simulink model "SF051A_SnsrOffsLrng"  (R2013b)
settings: Solver=FixedStepDiscrete  SolverMode=SingleTasking  StartTime=0.0  StopTime=1  FixedStep=0.002  RelTol=1e-3
undefined symbols (not defined in the file): ARCHGLBPRM_10MILLISEC_SEC_F32, ARCHGLBPRM_2MILLISEC_SEC_F32, ARCHGLBPRM_2PI_ULS_F32, ARCHGLBPRM_FLOATZEROTHD_ULS_F32, ARCHGLBPRM_PIOVER180_ULS_F32, CNV100MICROSECTOMILLISEC_MILLISECPERCNT_F32, CNV100MICROSECTOSEC_SECPERCNT_F32, COVRAMTRXNIT_ULS_F32, HWAUTHYTHD_ULS_F32, HWTQLRNGSTSLRND_CNT_U08, HWTQLRNGSTSNEGOFFS_CNT_U08, HWTQLRNGSTSNOTLRND_CNT_U08, HWTQLRNGSTSPOSOFFS_CNT_U08, HWTQLRNGSTSZEROOFFS_CNT_U08, HWTQLRNGTMRHILIM_SEC_F32, IDYMTRX_ULS_F32, IVS10MS_ULSPERSEC_F32, LRNGFILTICON_ULS_F32, NvmGetErrSts1, ONE_ULS_F32, SnsrOffsLrnd, SnsrOffsLrngFctEna, SnsrOffsLrngHwAgLrngDrvgDstThd, SnsrOffsLrngHwAgLrngEna, SnsrOffsLrngHwAgLrngHwVelThd, SnsrOffsLrngHwAgLrngSysTqThd, SnsrOffsLrngHwAgLrngSysTqThdMed, SnsrOffsLrngHwAgLrngSysTqThdTrustd, SnsrOffsLrngHwAgLrngSysTqThdWide, SnsrOffsLrngHwAgLrngTi, SnsrOffsLrngHwAgLrngVehSpdThd, SnsrOffsLrngHwAgLrngYawOffsDbnd, SnsrOffsLrngHwAgLrngYawRateThd, SnsrOffsLrngHwAgOffsLim, SnsrOffsLrngHwTqLrngEna, SnsrOffsLrngHwTqLrngEnaTiThd, SnsrOffsLrngHwTqLrngHwAgDbnd, SnsrOffsLrngHwTqLrngHwAgThd, SnsrOffsLrngHwTqLrngHwTqThd, SnsrOffsLrngHwTqLrngHwTqZeroOffsThd, SnsrOffsLrngHwTqLrngHwVelThd, SnsrOffsLrngHwTqLrngMeasTi, SnsrOffsLrngHwTqLrngMeasTiScar, SnsrOffsLrngHwTqLrngSampleImbThd1, SnsrOffsLrngHwTqLrngSampleImbThd2, SnsrOffsLrngHwTqLrngSampleThd1, SnsrOffsLrngHwTqLrngSampleThd2, SnsrOffsLrngHwTqLrngTiWghtCoeff, SnsrOffsLrngHwTqLrngVehSpdThd, SnsrOffsLrngHwTqOffsLim, SnsrOffsLrngSampleCntForHwTqLrngRst, SnsrOffsLrngTqInpDetnPwrEstimnThd, SnsrOffsLrngTqInpDetnSinGenrAmp, SnsrOffsLrngTqInpDetnSinGenrFrq, SnsrOffsLrngTqInpDetnStg1FilGain, SnsrOffsLrngTqInpDetnStg1WinSize, SnsrOffsLrngTqInpDetnStg2FilGainCen, SnsrOffsLrngTqInpDetnStg2FilGainDwn, SnsrOffsLrngTqInpDetnStg2FilGainUp, SnsrOffsLrngTqInpDetnStg2WinSize ... (+15)
libraries: Fil x34, FixdToFloat x17, FloatToFixd x16, NxtrLim x15, simulink x12, NxtrAbslt x12, NxtrNvM x8, NxtrMin x5, NxtrMath x3
(part 5 of 11)

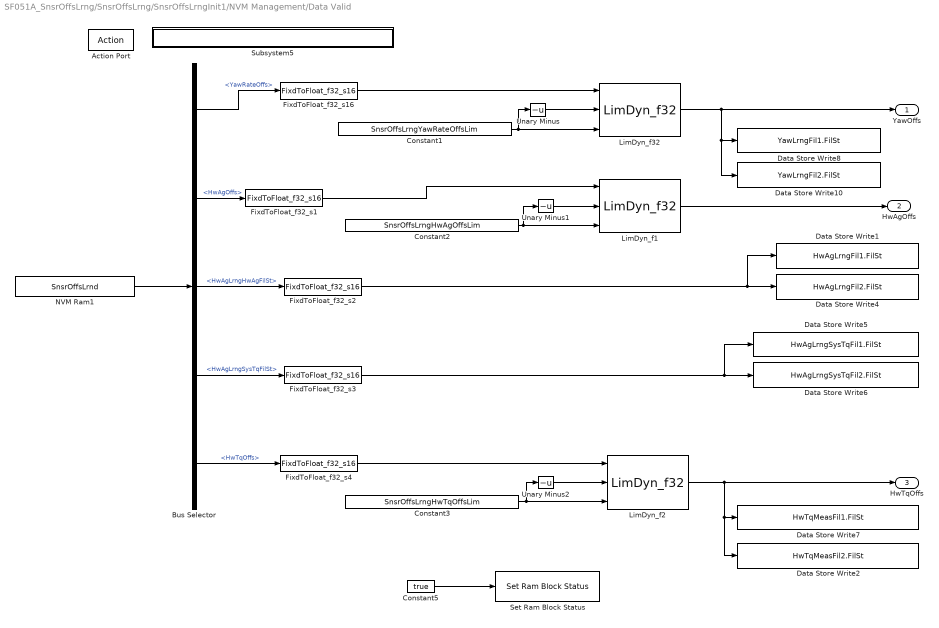
== system SF051A_SnsrOffsLrng/SnsrOffsLrng/SnsrOffsLrngInit1/NVM Management/Data Valid ==
  Action Port : ActionPort  ActionType=else
  Bus Selector : BusSelector  OutputSignals=YawRateOffs,HwAgOffs,HwAgLrngHwAgFilSt,HwAgLrngSysTqFilSt,HwTqOffs
  Constant1 : Constant  RequirementInfo={'linktype_rmi_doors' '0000babd (/E-STEER Core/SubSystem Specifications/Application Functions/SF051A Sensor Offset Learning)' '#SF051A_199' 'true' 'REQ:SF051A_199' '' } %GIDa_076ebffe_b680_48ef_8f96_8d7c4d22071c  Value=SnsrOffsLrngYawRateOffsLim  OutDataTypeStr=single
  Constant2 : Constant  RequirementInfo={'linktype_rmi_doors' '0000babd (/E-STEER Core/SubSystem Specifications/Application Functions/SF051A Sensor Offset Learning)' '#SF051A_200' 'true' 'REQ:SF051A_200' '' } %GIDa_86e1dd64_5744_4dce_ae9a_588dfe94c923  Value=SnsrOffsLrngHwAgOffsLim  OutDataTypeStr=single
  Constant3 : Constant  RequirementInfo={'linktype_rmi_doors' '0000babd (/E-STEER Core/SubSystem Specifications/Application Functions/SF051A Sensor Offset Learning)' '#SF051A_197' 'true' 'REQ:SF051A_197' '' } %GIDa_41a18de5_d6df_4abf_8798_f58c94a277e5  Value=SnsrOffsLrngHwTqOffsLim  OutDataTypeStr=single
  Constant5 : Constant  Value=true  OutDataTypeStr=boolean
      settings: AttributesFormatString=%<OutDataTypeStr>
  Data Store Write1 : DataStoreWrite  DataStoreName=HwAgLrngFil1  DataStoreElements=HwAgLrngFil1.FilSt
  Data Store Write10 : DataStoreWrite  DataStoreName=YawLrngFil2  DataStoreElements=YawLrngFil2.FilSt
  Data Store Write2 : DataStoreWrite  DataStoreName=HwTqMeasFil2  DataStoreElements=HwTqMeasFil2.FilSt
  Data Store Write4 : DataStoreWrite  DataStoreName=HwAgLrngFil2  DataStoreElements=HwAgLrngFil2.FilSt
  Data Store Write5 : DataStoreWrite  DataStoreName=HwAgLrngSysTqFil1  DataStoreElements=HwAgLrngSysTqFil1.FilSt
  Data Store Write6 : DataStoreWrite  DataStoreName=HwAgLrngSysTqFil2  DataStoreElements=HwAgLrngSysTqFil2.FilSt
  Data Store Write7 : DataStoreWrite  DataStoreName=HwTqMeasFil1  DataStoreElements=HwTqMeasFil1.FilSt
  Data Store Write8 : DataStoreWrite  DataStoreName=YawLrngFil1  DataStoreElements=YawLrngFil1.FilSt
  FixdToFloat_f32_s1 : FixdToFloat/FixdToFloat_f32_s16  Param1=10
  FixdToFloat_f32_s16 : FixdToFloat/FixdToFloat_f32_s16  Param1=9
  FixdToFloat_f32_s2 : FixdToFloat/FixdToFloat_f32_s16  Param1=4
  FixdToFloat_f32_s3 : FixdToFloat/FixdToFloat_f32_s16  Param1=5
  FixdToFloat_f32_s4 : FixdToFloat/FixdToFloat_f32_s16  Param1=12
  LimDyn_f1 : NxtrLim/LimDyn_f32  RequirementInfo={'linktype_rmi_doors' '0000babd (/E-STEER Core/SubSystem Specifications/Application Functions/SF051A Sensor Offset Learning)' '#SF051A_200' 'true' 'REQ:SF051A_200' '' } %GIDa_a6942d9b_ce75_427e_8670_f0f4de9cc18b
  LimDyn_f2 : NxtrLim/LimDyn_f32  RequirementInfo={'linktype_rmi_doors' '0000babd (/E-STEER Core/SubSystem Specifications/Application Functions/SF051A Sensor Offset Learning)' '#SF051A_197' 'true' 'REQ:SF051A_197' '' } %GIDa_a3cd0533_6baf_48d9_892e_aa8de74fd927
  LimDyn_f32 : NxtrLim/LimDyn_f32  RequirementInfo={'linktype_rmi_doors' '0000babd (/E-STEER Core/SubSystem Specifications/Application Functions/SF051A Sensor Offset Learning)' '#SF051A_199' 'true' 'REQ:SF051A_199' '' } %GIDa_1308976f_16df_4360_a216_3c89b58824fa
  NVM Ram1 : DataStoreRead  DataStoreName=SnsrOffsLrnd
  Set Ram Block Status : NxtrNvM/Set Ram Block Status  FuncName=Set Ram Block Status  NvMBlockName=SnsrOffsLrnd  VoidFuncRtn=on  BlockChanged_DSN=NvMSRBS_BlockChanged2  Return_DSN=NvMSRBS_Return2
      settings: AttributesFormatString=%<FuncName>
  Subsystem5 : Subsystem  Description=|  mask(Copyright Information){none=on}
      | Copyright info block.                                               
      |                                                                     
      | Place copyright information at the top of every subsystem in design.
      mask prompts: none "No parameters"
      mask help: Place copyright information at the top of every subsystem in design.
      mask Display:
      | NxtrConf = 'Nexteer Confidential';
      | 
      | sys = bdroot; %handle for the current model ("system")
      | first = get_param(sys,'Created');
      | first = first(end-3:end);  %year is last four digits
      | 
      | last = get_param(sys,'LastModifiedDate');
      | if isempty(last)
      |     last = datestr(now,'yyyy');
      | else
      |     last = last(end-3:end);
      | end
      | 
      | if strcmp(first,last)
      |     fprintf('%s -- Copyright %s Nexteer',NxtrConf,first)
      | else
      |     fprintf('%s -- %s%s- %s Nexteer',NxtrConf,char(169),first,last)
      | end
  Unary Minus : UnaryMinus  RequirementInfo={'linktype_rmi_doors' '0000babd (/E-STEER Core/SubSystem Specifications/Application Functions/SF051A Sensor Offset Learning)' '#SF051A_199' 'true' 'REQ:SF051A_199' '' } %GIDa_10d4a236_00c8_44d2_88c9_a38d910bd610
  Unary Minus1 : UnaryMinus  RequirementInfo={'linktype_rmi_doors' '0000babd (/E-STEER Core/SubSystem Specifications/Application Functions/SF051A Sensor Offset Learning)' '#SF051A_200' 'true' 'REQ:SF051A_200' '' } %GIDa_5c1b3055_1216_4150_a142_355401d5d7f1
  Unary Minus2 : UnaryMinus  RequirementInfo={'linktype_rmi_doors' '0000babd (/E-STEER Core/SubSystem Specifications/Application Functions/SF051A Sensor Offset Learning)' '#SF051A_197' 'true' 'REQ:SF051A_197' '' } %GIDa_8a9aa98b_e7a9_4fa6_add4_1fe4b896ad88
  YawOffs : Outport
  HwAgOffs : Outport  Port=2
  HwTqOffs : Outport  Port=3
  wires:
  NVM Ram1/1 -> Bus Selector/1
  Bus Selector/1 -> FixdToFloat_f32_s16/1  "<YawRateOffs>"
  Bus Selector/2 -> FixdToFloat_f32_s1/1  "<HwAgOffs>"
  Bus Selector/5 -> FixdToFloat_f32_s4/1  "<HwTqOffs>"
  Constant1/1 -> LimDyn_f32/3, Unary Minus/1
  LimDyn_f32/1 -> YawOffs/1, Data Store Write8/1, Data Store Write10/1
  Constant2/1 -> Unary Minus1/1, LimDyn_f1/3
  Constant3/1 -> Unary Minus2/1, LimDyn_f2/3
  LimDyn_f2/1 -> Data Store Write2/1, Data Store Write7/1, HwTqOffs/1
  Bus Selector/4 -> FixdToFloat_f32_s3/1  "<HwAgLrngSysTqFilSt>"
  Bus Selector/3 -> FixdToFloat_f32_s2/1  "<HwAgLrngHwAgFilSt>"
  Constant5/1 -> Set Ram Block Status/1
  FixdToFloat_f32_s2/1 -> Data Store Write1/1, Data Store Write4/1
  FixdToFloat_f32_s3/1 -> Data Store Write5/1, Data Store Write6/1
  Unary Minus/1 -> LimDyn_f32/2
  Unary Minus2/1 -> LimDyn_f2/2
  FixdToFloat_f32_s4/1 -> LimDyn_f2/1
  FixdToFloat_f32_s16/1 -> LimDyn_f32/1
  LimDyn_f1/1 -> HwAgOffs/1
  Unary Minus1/1 -> LimDyn_f1/2
  FixdToFloat_f32_s1/1 -> LimDyn_f1/1

== system SF051A_SnsrOffsLrng/SnsrOffsLrng/SnsrOffsLrngInit1/NVM Management/Not Enabled ==
  note: The entire function has been disabled via one boolean calibration.  Output zeros
      | and tell Nvm Mgr not to bother writing Nvm values at key off.
  Action Port : ActionPort  ActionType=then
  Constant : Constant  RequirementInfo={'linktype_rmi_doors' '0000babd (/E-STEER Core/SubSystem Specifications/Application Functions/SF051A Sensor Offset Learning)' '#SF051A_244' 'true' 'REQ:SF051A_244' '' ; 'linktype_rmi_doors' '0000babd (/E-STEER Core/SubSystem Specifications/Application Functions/SF051A Sensor Offset Learning)' '#SF051A_245' 'true' 'REQ:SF051A_245' '' ; 'linktype_rmi_doors' '0000babd (/E-STEER Core/SubSystem Specifications/Application Functions/SF051A Sensor Offset Learning)' '#SF051A_45' 'true' 'REQ:SF051A_45' '' } %GIDa_7bd904ef_6dfb_4655_9af9_edb8e6d91ac1  Value=ZERO_ULS_F32  OutDataTypeStr=single
      settings: AttributesFormatString=%<OutDataTypeStr>
  Subsystem5 : Subsystem  Description=|  mask(Copyright Information){none=on}
      | Copyright info block.                                               
      |                                                                     
      | Place copyright information at the top of every subsystem in design.
      mask prompts: none "No parameters"
      mask help: Place copyright information at the top of every subsystem in design.
      mask Display:
      | NxtrConf = 'Nexteer Confidential';
      | 
      | sys = bdroot; %handle for the current model ("system")
      | first = get_param(sys,'Created');
      | first = first(end-3:end);  %year is last four digits
      | 
      | last = get_param(sys,'LastModifiedDate');
      | if isempty(last)
      |     last = datestr(now,'yyyy');
      | else
      |     last = last(end-3:end);
      | end
      | 
      | if strcmp(first,last)
      |     fprintf('%s -- Copyright %s Nexteer',NxtrConf,first)
      | else
      |     fprintf('%s -- %s%s- %s Nexteer',NxtrConf,char(169),first,last)
      | end
  YawOffs : Outport  RequirementInfo={'linktype_rmi_doors' '0000babd (/E-STEER Core/SubSystem Specifications/Application Functions/SF051A Sensor Offset Learning)' '#SF051A_244' 'true' 'REQ:SF051A_244' '' } %GIDa_19bbba3b_0dec_46be_8ce3_0daa8b4bfd81
  HwAgOffs : Outport  RequirementInfo={'linktype_rmi_doors' '0000babd (/E-STEER Core/SubSystem Specifications/Application Functions/SF051A Sensor Offset Learning)' '#SF051A_245' 'true' 'REQ:SF051A_245' '' } %GIDa_7ded515a_2b55_49df_86d7_0efec96a218f  Port=2
  HwTqOffs : Outport  RequirementInfo={'linktype_rmi_doors' '0000babd (/E-STEER Core/SubSystem Specifications/Application Functions/SF051A Sensor Offset Learning)' '#SF051A_45' 'true' 'REQ:SF051A_45' '' } %GIDa_401e0381_36a7_4d73_9c61_1f70a1280659  Port=3
  wires:
  Constant/1 -> HwTqOffs/1, HwAgOffs/1, YawOffs/1

== system SF051A_SnsrOffsLrng/SnsrOffsLrng/SnsrOffsLrngInit1/NVM Management/Subsystem5 ==

== system SF051A_SnsrOffsLrng/SnsrOffsLrng/SnsrOffsLrngPer1/EnableLearning/Default_TqInpDetn ==
  Action Port : ActionPort  ActionType=else
  Constant : Constant  Value=false  OutDataTypeStr=boolean
      settings: AttributesFormatString=%<OutDataTypeStr>
  Constant1 : Constant  Value=true  OutDataTypeStr=boolean
      settings: AttributesFormatString=%<OutDataTypeStr>
  Subsystem5 : Subsystem  Description=|  mask(Copyright Information){none=on}
      | Copyright info block.                                               
      |                                                                     
      | Place copyright information at the top of every subsystem in design.
      mask prompts: none "No parameters"
      mask help: Place copyright information at the top of every subsystem in design.
      mask Display:
      | NxtrConf = 'Nexteer Confidential';
      | 
      | sys = bdroot; %handle for the current model ("system")
      | first = get_param(sys,'Created');
      | first = first(end-3:end);  %year is last four digits
      | 
      | last = get_param(sys,'LastModifiedDate');
      | if isempty(last)
      |     last = datestr(now,'yyyy');
      | else
      |     last = last(end-3:end);
      | end
      | 
      | if strcmp(first,last)
      |     fprintf('%s -- Copyright %s Nexteer',NxtrConf,first)
      | else
      |     fprintf('%s -- %s%s- %s Nexteer',NxtrConf,char(169),first,last)
      | end
  TqInpPresVld : Outport  InitialOutput=0
  TqInpPrsnt : Outport  Port=2  InitialOutput=0
  wires:
  Constant1/1 -> TqInpPrsnt/1  "TqInpPrsnt"
  Constant/1 -> TqInpPresVld/1  "TqInpPresVld"

== system SF051A_SnsrOffsLrng/SnsrOffsLrng/SnsrOffsLrngPer1/EnableLearning/EnablingConditions ==
  note: Prevents to keep taking the same measurements once again
      | again if the handwheel didn't chaged its position
  note: Limits the HwPos range that will be used for the learning.
      | defined by the Learning algorithm
  note: Vehicle speed need to be 0 kph in order to get less noisy
      | measurements. It is also the situation when it is most probable
      | to find a NoTorqueInputPresent situation.
  note: Handwheel need to be stopped.
  note: Handwheel torque needs to be close to zero.. This claibration
      | cannot have the same value than the maximum HwTrq that
      | will be stored (Learning algotihm needs HwTrq values out of that
      | range in order to work).
  HwTq : Inport
  HwVel : Inport  Port=2
  VehSpd : Inport  Port=3
  HwAg : Inport  Port=4
  Abslt_f32_f1 : NxtrAbslt/Abslt_f32_f32  RequirementInfo={'linktype_rmi_doors' '0000babd (/E-STEER Core/SubSystem Specifications/Application Functions/SF051A Sensor Offset Learning)' '#SF051A_164' 'true' 'REQ:SF051A_164' '' } %GIDa_9e6654fc_c12f_4f0b_b95d_e68a683dad8f  SFunctionSpec=single y1 = Abslt_f32_f32(single u1)
      settings: AttributesFormatString=%<Name>
  Abslt_f32_f2 : NxtrAbslt/Abslt_f32_f32  RequirementInfo={'linktype_rmi_doors' '0000babd (/E-STEER Core/SubSystem Specifications/Application Functions/SF051A Sensor Offset Learning)' '#SF051A_164' 'true' 'REQ:SF051A_164' '' } %GIDa_f22554bc_685a_43e5_b318_a11f967165d9  SFunctionSpec=single y1 = Abslt_f32_f32(single u1)
      settings: AttributesFormatString=%<Name>
  Abslt_f32_f32 : NxtrAbslt/Abslt_f32_f32  RequirementInfo={'linktype_rmi_doors' '0000babd (/E-STEER Core/SubSystem Specifications/Application Functions/SF051A Sensor Offset Learning)' '#SF051A_164' 'true' 'REQ:SF051A_164' '' } %GIDa_e92dafa2_36c7_4571_935e_c15c4f7f6a46  SFunctionSpec=single y1 = Abslt_f32_f32(single u1)
      settings: AttributesFormatString=%<Name>
  CheckLastMeasHwPos : Subsystem  RequirementInfo={'linktype_rmi_doors' '0000babd (/E-STEER Core/SubSystem Specifications/Application Functions/SF051A Sensor Offset Learning)' '#SF051A_153' 'true' 'REQ:SF051A_153' '' } %GIDa_44e6e44d_9c2d_4a29_b17b_bdb322509a04
  Constant : Constant  RequirementInfo={'linktype_rmi_doors' '0000babd (/E-STEER Core/SubSystem Specifications/Application Functions/SF051A Sensor Offset Learning)' '#SF051A_164' 'true' 'REQ:SF051A_164' '' } %GIDa_78b0b28d_512c_4bbe_9a88_b290db340ca2  Value=SnsrOffsLrngHwTqLrngHwTqThd
  Constant1 : Constant  RequirementInfo={'linktype_rmi_doors' '0000babd (/E-STEER Core/SubSystem Specifications/Application Functions/SF051A Sensor Offset Learning)' '#SF051A_164' 'true' 'REQ:SF051A_164' '' } %GIDa_6cae68dc_855b_480e_9fca_bfbaa07e5595  Value=SnsrOffsLrngHwTqLrngHwVelThd
  Constant2 : Constant  RequirementInfo={'linktype_rmi_doors' '0000babd (/E-STEER Core/SubSystem Specifications/Application Functions/SF051A Sensor Offset Learning)' '#SF051A_164' 'true' 'REQ:SF051A_164' '' } %GIDa_db8aa412_af43_4293_866b_dc91b376e004  Value=SnsrOffsLrngHwTqLrngVehSpdThd
  Constant3 : Constant  RequirementInfo={'linktype_rmi_doors' '0000babd (/E-STEER Core/SubSystem Specifications/Application Functions/SF051A Sensor Offset Learning)' '#SF051A_164' 'true' 'REQ:SF051A_164' '' } %GIDa_56d7e85f_b29d_46f1_86ec_479da9e5d3a2  Value=SnsrOffsLrngHwTqLrngHwAgThd
  Logical Operator : Logic  RequirementInfo={'linktype_rmi_doors' '0000babd (/E-STEER Core/SubSystem Specifications/Application Functions/SF051A Sensor Offset Learning)' '#SF051A_164' 'true' 'REQ:SF051A_164' '' ; 'linktype_rmi_doors' '0000babd (/E-STEER Core/SubSystem Specifications/Application Functions/SF051A Sensor Offset Learning)' '#SF051A_153' 'true' 'REQ:SF051A_153' '' } %GIDa_67f5e3c6_c811_4f06_9205_8d434655c309  Inputs=5  AllPortsSameDT=off  OutDataTypeStr=boolean
  Relational Operator : RelationalOperator  RequirementInfo={'linktype_rmi_doors' '0000babd (/E-STEER Core/SubSystem Specifications/Application Functions/SF051A Sensor Offset Learning)' '#SF051A_164' 'true' 'REQ:SF051A_164' '' } %GIDa_64107afe_b0ad_4ff5_abd5_e1ad1dd60b07  Operator=<=  OutDataTypeStr=boolean
  Relational Operator1 : RelationalOperator  RequirementInfo={'linktype_rmi_doors' '0000babd (/E-STEER Core/SubSystem Specifications/Application Functions/SF051A Sensor Offset Learning)' '#SF051A_164' 'true' 'REQ:SF051A_164' '' } %GIDa_a80d4eac_68b4_4a5c_93ef_0c10081c4193  Operator=<=  OutDataTypeStr=boolean
  Relational Operator2 : RelationalOperator  RequirementInfo={'linktype_rmi_doors' '0000babd (/E-STEER Core/SubSystem Specifications/Application Functions/SF051A Sensor Offset Learning)' '#SF051A_164' 'true' 'REQ:SF051A_164' '' } %GIDa_b1b96eb6_2e47_4324_bb24_5b2841330fb5  Operator=<=  OutDataTypeStr=boolean
  Relational Operator3 : RelationalOperator  RequirementInfo={'linktype_rmi_doors' '0000babd (/E-STEER Core/SubSystem Specifications/Application Functions/SF051A Sensor Offset Learning)' '#SF051A_164' 'true' 'REQ:SF051A_164' '' } %GIDa_3484eb6c_a506_422c_9fce_52f4631db782  Operator=<=  OutDataTypeStr=boolean
  Subsystem5 : Subsystem  Description=|  mask(Copyright Information){none=on}
      | Copyright info block.                                               
      |                                                                     
      | Place copyright information at the top of every subsystem in design.
      mask prompts: none "No parameters"
      mask help: Place copyright information at the top of every subsystem in design.
      mask Display:
      | NxtrConf = 'Nexteer Confidential';
      | 
      | sys = bdroot; %handle for the current model ("system")
      | first = get_param(sys,'Created');
      | first = first(end-3:end);  %year is last four digits
      | 
      | last = get_param(sys,'LastModifiedDate');
      | if isempty(last)
      |     last = datestr(now,'yyyy');
      | else
      |     last = last(end-3:end);
      | end
      | 
      | if strcmp(first,last)
      |     fprintf('%s -- Copyright %s Nexteer',NxtrConf,first)
      | else
      |     fprintf('%s -- %s%s- %s Nexteer',NxtrConf,char(169),first,last)
      | end
  TqInpDetnEna : Outport
  wires:
  CheckLastMeasHwPos/1(HwAgMoved) -> Logical Operator/5
  Abslt_f32_f2/1 -> Relational Operator3/1
  Constant3/1 -> Relational Operator3/2
  VehSpd/1 -> Relational Operator2/1
  Constant2/1 -> Relational Operator2/2
  Abslt_f32_f1/1 -> Relational Operator1/1
  Constant1/1 -> Relational Operator1/2
  Constant/1 -> Relational Operator/2
  Abslt_f32_f32/1 -> Relational Operator/1
  Relational Operator3/1 -> Logical Operator/4
  HwAg/1 -> Abslt_f32_f2/1, CheckLastMeasHwPos/1(HwAg)
  Logical Operator/1 -> TqInpDetnEna/1  "TqInpDetnEna"
  Relational Operator1/1 -> Logical Operator/2
  HwVel/1 -> Abslt_f32_f1/1
  HwTq/1 -> Abslt_f32_f32/1
  Relational Operator2/1 -> Logical Operator/3
  Relational Operator/1 -> Logical Operator/1

== system SF051A_SnsrOffsLrng/SnsrOffsLrng/SnsrOffsLrngPer1/EnableLearning/Eval_Time ==
  note: In MilliSec
  Action Port : ActionPort  ActionType=then
  100MicroSecToMilliSec : Constant  Value=CNV100MICROSECTOMILLISEC_MILLISECPERCNT_F32
  Constant : Constant  Value=SnsrOffsLrngHwTqLrngEnaTiThd
  Data Store Read : DataStoreRead  DataStoreName=HwTqLrngEnaTmrRef
  FixdToFloat_f32_u32 : FixdToFloat/FixdToFloat_f32_u32  Param1=0
  GetTiSpan100MicroSec32bit : Subsystem  mask(Timer_GTS){}
      mask help: Used to get the time span between start and current time.
  Product : Product
  Relational Operator : RelationalOperator  OutDataTypeStr=boolean
  Subsystem5 : Subsystem  Description=|  mask(Copyright Information){none=on}
      | Copyright info block.                                               
      |                                                                     
      | Place copyright information at the top of every subsystem in design.
      mask prompts: none "No parameters"
      mask help: Place copyright information at the top of every subsystem in design.
      mask Display:
      | NxtrConf = 'Nexteer Confidential';
      | 
      | sys = bdroot; %handle for the current model ("system")
      | first = get_param(sys,'Created');
      | first = first(end-3:end);  %year is last four digits
      | 
      | last = get_param(sys,'LastModifiedDate');
      | if isempty(last)
      |     last = datestr(now,'yyyy');
      | else
      |     last = last(end-3:end);
      | end
      | 
      | if strcmp(first,last)
      |     fprintf('%s -- Copyright %s Nexteer',NxtrConf,first)
      | else
      |     fprintf('%s -- %s%s- %s Nexteer',NxtrConf,char(169),first,last)
      | end
  HwTqLrngEna : Outport
  wires:
  Data Store Read/1 -> GetTiSpan100MicroSec32bit/1(RefTmr)
  Constant/1 -> Relational Operator/2
  Relational Operator/1 -> HwTqLrngEna/1
  GetTiSpan100MicroSec32bit/1(TiSpan) -> FixdToFloat_f32_u32/1
  Product/1 -> Relational Operator/1
  100MicroSecToMilliSec/1 -> Product/2
  FixdToFloat_f32_u32/1 -> Product/1

== system SF051A_SnsrOffsLrng/SnsrOffsLrng/SnsrOffsLrngPer1/EnableLearning/False_Reset ==
  Action Port : ActionPort  ActionType=else
  Constant : Constant  Value=false  OutDataTypeStr=boolean
      settings: AttributesFormatString=%<OutDataTypeStr>
  Data Store Write : DataStoreWrite  DataStoreName=HwTqLrngEnaTmrRef
  GetRefTmr100MicroSec32bit : Subsystem
  Subsystem5 : Subsystem  Description=|  mask(Copyright Information){none=on}
      | Copyright info block.                                               
      |                                                                     
      | Place copyright information at the top of every subsystem in design.
      mask prompts: none "No parameters"
      mask help: Place copyright information at the top of every subsystem in design.
      mask Display:
      | NxtrConf = 'Nexteer Confidential';
      | 
      | sys = bdroot; %handle for the current model ("system")
      | first = get_param(sys,'Created');
      | first = first(end-3:end);  %year is last four digits
      | 
      | last = get_param(sys,'LastModifiedDate');
      | if isempty(last)
      |     last = datestr(now,'yyyy');
      | else
      |     last = last(end-3:end);
      | end
      | 
      | if strcmp(first,last)
      |     fprintf('%s -- Copyright %s Nexteer',NxtrConf,first)
      | else
      |     fprintf('%s -- %s%s- %s Nexteer',NxtrConf,char(169),first,last)
      | end
  HwTqLrngEna : Outport
  wires:
  Constant/1 -> HwTqLrngEna/1
  GetRefTmr100MicroSec32bit/1(RefTmr) -> Data Store Write/1

== system SF051A_SnsrOffsLrng/SnsrOffsLrng/SnsrOffsLrngPer1/EnableLearning/Filter_HwTq ==
  HwTq : Inport
  Display : DataStoreWrite  DataStoreName=dSnsrOffsLrngTqInpDetnHwTqFild
  FilLpUpdOutp : Fil/FilLpUpdOutp  StVar=TqInpDetnHwTqFil
      settings: AttributesFormatString=StVar: %<StVar>
  Subsystem5 : Subsystem  Description=|  mask(Copyright Information){none=on}
      | Copyright info block.                                               
      |                                                                     
      | Place copyright information at the top of every subsystem in design.
      mask prompts: none "No parameters"
      mask help: Place copyright information at the top of every subsystem in design.
      mask Display:
      | NxtrConf = 'Nexteer Confidential';
      | 
      | sys = bdroot; %handle for the current model ("system")
      | first = get_param(sys,'Created');
      | first = first(end-3:end);  %year is last four digits
      | 
      | last = get_param(sys,'LastModifiedDate');
      | if isempty(last)
      |     last = datestr(now,'yyyy');
      | else
      |     last = last(end-3:end);
      | end
      | 
      | if strcmp(first,last)
      |     fprintf('%s -- Copyright %s Nexteer',NxtrConf,first)
      | else
      |     fprintf('%s -- %s%s- %s Nexteer',NxtrConf,char(169),first,last)
      | end
  HwTqFild : Outport
  wires:
  HwTq/1 -> FilLpUpdOutp/1
  FilLpUpdOutp/1 -> Display/1, HwTqFild/1

== system SF051A_SnsrOffsLrng/SnsrOffsLrng/SnsrOffsLrngPer1/EnableLearning/Perform_TqInpDetn ==
  note: Reset may or may not happen, but if it does, it must happen before PreProcessing executes.
  note: Step 1
  note: Step 2
  HwTqFild : Inport
  TqInpDetnEnaPrev : Inport  Port=2
  Action Port : ActionPort  ActionType=then
  Do nothing : Subsystem  TreatAsAtomicUnit=on
  ElapsedTime : Subsystem  Priority=2
      settings: AttributesFormatString=Priority: %<Priority>
  Enable_PreProcessing : Subsystem  Priority=2  TreatAsAtomicUnit=on
      settings: AttributesFormatString=Priority: %<Priority>
  If1 : If  Priority=1  IfExpression=~u1
      settings: AttributesFormatString=Priority: %<Priority>
  SetStuffToZero : Subsystem  Priority=1  TreatAsAtomicUnit=on
      settings: AttributesFormatString=Priority: %<Priority>
  StateVariable : DataStoreWrite  Priority=2  DataStoreName=HwTqLrngTqInpPrsnt
      settings: AttributesFormatString=Priority: %<Priority>
  Subsystem5 : Subsystem  Description=|  mask(Copyright Information){none=on}
      | Copyright info block.                                               
      |                                                                     
      | Place copyright information at the top of every subsystem in design.
      mask prompts: none "No parameters"
      mask help: Place copyright information at the top of every subsystem in design.
      mask Display:
      | NxtrConf = 'Nexteer Confidential';
      | 
      | sys = bdroot; %handle for the current model ("system")
      | first = get_param(sys,'Created');
      | first = first(end-3:end);  %year is last four digits
      | 
      | last = get_param(sys,'LastModifiedDate');
      | if isempty(last)
      |     last = datestr(now,'yyyy');
      | else
      |     last = last(end-3:end);
      | end
      | 
      | if strcmp(first,last)
      |     fprintf('%s -- Copyright %s Nexteer',NxtrConf,first)
      | else
      |     fprintf('%s -- %s%s- %s Nexteer',NxtrConf,char(169),first,last)
      | end
  TqInpPrsntVld : Outport  InitialOutput=0
  TqInpPrsnt : Outport  Port=2  InitialOutput=0
  wires:
  ElapsedTime/1(TiEnad) -> Enable_PreProcessing/1(TiEnad)
  Enable_PreProcessing/2(TqInpPrsnt) -> TqInpPrsnt/1, StateVariable/1  "TqInpPrsnt"
  Enable_PreProcessing/1(TqInpPrsntVld) -> TqInpPrsntVld/1  "TqInpPrsntVld"
  If1/1 -> SetStuffToZero/Action
  TqInpDetnEnaPrev/1 -> If1/1
  HwTqFild/1 -> Enable_PreProcessing/2(HwTqFild)
  If1/2 -> Do nothing/Action

== system SF051A_SnsrOffsLrng/SnsrOffsLrng/SnsrOffsLrngPer1/EnableLearning/Subsystem5 ==

== system SF051A_SnsrOffsLrng/SnsrOffsLrng/SnsrOffsLrngPer1/Hold/Subsystem5 ==

== system SF051A_SnsrOffsLrng/SnsrOffsLrng/SnsrOffsLrngPer1/Learning/CalculateOnCenterTorqueDrift ==
  note: The considered mathematical model HwTq vs HwAg follows:
      |                    Y = A*sin(X + Phi) + B
      | Where:
      | -. X = HwAg
      | -. Y = HwTq
      | -. A is the HwTq reading when Tq_Off=0Nm, Phi=0Deg and HwAg=90°
      | -. Phi = HwAg_Offset
      | -. B = HwTq_Offset
      |
      | That model can also be written as:
      |                Y = A1*sin(X) + A2*cos(X) + B
      | Where: A = sqrt(A1^2+A2^2)   and   sin(Phi) = A2/A
      |
      | The RLSE estimates the parameters A1, A2 and B, which are used to
      | calculate the HwTq Offset.
  note: In this version, the HwTq Offset is considered more specifically as the
      | HwTq drift for HwAg = 0Deg (OnCenter). Replacing in the mathematical
      | model:
      |                Y = A1*sin(0°) + A2*cos(0°) + B
      |                             Y = A2 + B
      | Therefore,
      |           HwTqOnCenterDrift = A2 + HwTq_Off
  HwTqOffsEstimd : Inport
  A2 : Inport  Port=2
  Add1 : Sum
  Display1 : DataStoreWrite  DataStoreName=dSnsrOffsLrngHwTqLrngHwTqOffsRaw
  Subsystem5 : Subsystem  Description=|  mask(Copyright Information){none=on}
      | Copyright info block.                                               
      |                                                                     
      | Place copyright information at the top of every subsystem in design.
      mask prompts: none "No parameters"
      mask help: Place copyright information at the top of every subsystem in design.
      mask Display:
      | NxtrConf = 'Nexteer Confidential';
      | 
      | sys = bdroot; %handle for the current model ("system")
      | first = get_param(sys,'Created');
      | first = first(end-3:end);  %year is last four digits
      | 
      | last = get_param(sys,'LastModifiedDate');
      | if isempty(last)
      |     last = datestr(now,'yyyy');
      | else
      |     last = last(end-3:end);
      | end
      | 
      | if strcmp(first,last)
      |     fprintf('%s -- Copyright %s Nexteer',NxtrConf,first)
      | else
      |     fprintf('%s -- %s%s- %s Nexteer',NxtrConf,char(169),first,last)
      | end
  HwTqDriftEstimnOnCentr : Outport
  wires:
  A2/1 -> Add1/1
  HwTqOffsEstimd/1 -> Add1/2
  Add1/1 -> Display1/1, HwTqDriftEstimnOnCentr/1

== system SF051A_SnsrOffsLrng/SnsrOffsLrng/SnsrOffsLrngPer1/Learning/Counter ==
  note: 0 is considered positive
  HwAgMeasd : Inport  RequirementInfo={'linktype_rmi_doors' '0000babd (/E-STEER Core/SubSystem Specifications/Application Functions/SF051A Sensor Offset Learning)' '#SF051A_178' 'true' 'REQ:SF051A_178' '' ; 'linktype_rmi_doors' '0000babd (/E-STEER Core/SubSystem Specifications/Application Functions/SF051A Sensor Offset Learning)' '#SF051A_180' 'true' 'REQ:SF051A_180' '' } %GIDa_0b7cbbdd_6749_44e6_8c03_3d3beeb58276
  Add : Sum  RequirementInfo={'linktype_rmi_doors' '0000babd (/E-STEER Core/SubSystem Specifications/Application Functions/SF051A Sensor Offset Learning)' '#SF051A_177' 'true' 'REQ:SF051A_177' '' } %GIDa_5eff4b52_c2be_4a1c_aa45_1e5de2bd3d72
  Constant : Constant  RequirementInfo={'linktype_rmi_doors' '0000babd (/E-STEER Core/SubSystem Specifications/Application Functions/SF051A Sensor Offset Learning)' '#SF051A_180' 'true' 'REQ:SF051A_180' '' ; 'linktype_rmi_doors' '0000babd (/E-STEER Core/SubSystem Specifications/Application Functions/SF051A Sensor Offset Learning)' '#SF051A_178' 'true' 'REQ:SF051A_178' '' } %GIDa_539e9637_0cf6_41e3_a23a_bb72c667b607  Value=ZERO_ULS_F32  OutDataTypeStr=single
      settings: AttributesFormatString=%<OutDataTypeStr>
  Data Type Conversion : DataTypeConversion  OutDataTypeStr=single
  Data Type Conversion1 : DataTypeConversion  OutDataTypeStr=single
  Display1 : DataStoreWrite  DataStoreName=dSnsrOffsLrngHwTqLrngSampleCntTot
  If : If  RequirementInfo={'linktype_rmi_doors' '0000babd (/E-STEER Core/SubSystem Specifications/Application Functions/SF051A Sensor Offset Learning)' '#SF051A_180' 'true' 'REQ:SF051A_180' '' ; 'linktype_rmi_doors' '0000babd (/E-STEER Core/SubSystem Specifications/Application Functions/SF051A Sensor Offset Learning)' '#SF051A_178' 'true' 'REQ:SF051A_178' '' } %GIDa_b0392e2d_651d_4636_962e_93d698ea8f42  IfExpression=u1
  Increment_SampleCntNeg : Subsystem  RequirementInfo={'linktype_rmi_doors' '0000babd (/E-STEER Core/SubSystem Specifications/Application Functions/SF051A Sensor Offset Learning)' '#SF051A_178' 'true' 'REQ:SF051A_178' '' } %GIDa_afa173dc_df46_47f6_a45c_3e401303be1d  TreatAsAtomicUnit=on
  Increment_SampleCntPos : Subsystem  RequirementInfo={'linktype_rmi_doors' '0000babd (/E-STEER Core/SubSystem Specifications/Application Functions/SF051A Sensor Offset Learning)' '#SF051A_180' 'true' 'REQ:SF051A_180' '' } %GIDa_1266e2e5_d133_412e_8403_c3567846effb  TreatAsAtomicUnit=on
  Relational Operator : RelationalOperator  RequirementInfo={'linktype_rmi_doors' '0000babd (/E-STEER Core/SubSystem Specifications/Application Functions/SF051A Sensor Offset Learning)' '#SF051A_180' 'true' 'REQ:SF051A_180' '' ; 'linktype_rmi_doors' '0000babd (/E-STEER Core/SubSystem Specifications/Application Functions/SF051A Sensor Offset Learning)' '#SF051A_178' 'true' 'REQ:SF051A_178' '' } %GIDa_66c0a436_7235_4f62_8876_d110de8c5c01  OutDataTypeStr=boolean
  Subsystem5 : Subsystem  Description=|  mask(Copyright Information){none=on}
      | Copyright info block.                                               
      |                                                                     
      | Place copyright information at the top of every subsystem in design.
      mask prompts: none "No parameters"
      mask help: Place copyright information at the top of every subsystem in design.
      mask Display:
      | NxtrConf = 'Nexteer Confidential';
      | 
      | sys = bdroot; %handle for the current model ("system")
      | first = get_param(sys,'Created');
      | first = first(end-3:end);  %year is last four digits
      | 
      | last = get_param(sys,'LastModifiedDate');
      | if isempty(last)
      |     last = datestr(now,'yyyy');
      | else
      |     last = last(end-3:end);
      | end
      | 
      | if strcmp(first,last)
      |     fprintf('%s -- Copyright %s Nexteer',NxtrConf,first)
      | else
      |     fprintf('%s -- %s%s- %s Nexteer',NxtrConf,char(169),first,last)
      | end
  SampleCntTot : Outport  OutDataTypeStr=single
  SampleCntPos : Outport  Port=2  OutDataTypeStr=single
  SampleCntNeg : Outport  Port=3  OutDataTypeStr=single
  wires:
  If/1 -> Increment_SampleCntPos/Action
  If/2 -> Increment_SampleCntNeg/Action
  Increment_SampleCntPos/1(Size) -> Data Type Conversion/1
  Increment_SampleCntNeg/1(Size) -> Data Type Conversion1/1
  Add/1 -> Display1/1, SampleCntTot/1
  Data Type Conversion/1 -> Add/1, SampleCntPos/1
  Data Type Conversion1/1 -> Add/2, SampleCntNeg/1
  HwAgMeasd/1 -> Relational Operator/1
  Relational Operator/1 -> If/1
  Constant/1 -> Relational Operator/2

== system SF051A_SnsrOffsLrng/SnsrOffsLrng/SnsrOffsLrngPer1/Learning/Do nothing ==
  Action Port : ActionPort  ActionType=else
  Subsystem5 : Subsystem  Description=|  mask(Copyright Information){none=on}
      | Copyright info block.                                               
      |                                                                     
      | Place copyright information at the top of every subsystem in design.
      mask prompts: none "No parameters"
      mask help: Place copyright information at the top of every subsystem in design.
      mask Display:
      | NxtrConf = 'Nexteer Confidential';
      | 
      | sys = bdroot; %handle for the current model ("system")
      | first = get_param(sys,'Created');
      | first = first(end-3:end);  %year is last four digits
      | 
      | last = get_param(sys,'LastModifiedDate');
      | if isempty(last)
      |     last = datestr(now,'yyyy');
      | else
      |     last = last(end-3:end);
      | end
      | 
      | if strcmp(first,last)
      |     fprintf('%s -- Copyright %s Nexteer',NxtrConf,first)
      | else
      |     fprintf('%s -- %s%s- %s Nexteer',NxtrConf,char(169),first,last)
      | end

== system SF051A_SnsrOffsLrng/SnsrOffsLrng/SnsrOffsLrngPer1/Learning/ForgettingFactor ==
  SampleCntTot : Inport  RequirementInfo={'linktype_rmi_doors' '0000babd (/E-STEER Core/SubSystem Specifications/Application Functions/SF051A Sensor Offset Learning)' '#SF051A_243' 'true' 'REQ:SF051A_243' '' } %GIDa_3a0dab8d_8899_4510_9d33_ef745ce09e6f
  Constant1 : Constant  RequirementInfo={'linktype_rmi_doors' '0000babd (/E-STEER Core/SubSystem Specifications/Application Functions/SF051A Sensor Offset Learning)' '#SF051A_243' 'true' 'REQ:SF051A_243' '' } %GIDa_21d51c87_7466_4d2f_9d56_8aff611e59ee  Value=SnsrOffsLrngSampleCntForHwTqLrngRst  OutDataTypeStr=uint16
      settings: AttributesFormatString=%<OutDataTypeStr>
  Data Type Conversion : DataTypeConversion  RequirementInfo={'linktype_rmi_doors' '0000babd (/E-STEER Core/SubSystem Specifications/Application Functions/SF051A Sensor Offset Learning)' '#SF051A_243' 'true' 'REQ:SF051A_243' '' } %GIDa_34adf385_e0dc_4431_ad93_b255baa8cd9d  OutDataTypeStr=uint16
  If : If  RequirementInfo={'linktype_rmi_doors' '0000babd (/E-STEER Core/SubSystem Specifications/Application Functions/SF051A Sensor Offset Learning)' '#SF051A_243' 'true' 'REQ:SF051A_243' '' } %GIDa_00ffddbc_2a9f_416d_92ac_8237a6566e70  IfExpression=u1  ShowElse=off
  Relational Operator1 : RelationalOperator  RequirementInfo={'linktype_rmi_doors' '0000babd (/E-STEER Core/SubSystem Specifications/Application Functions/SF051A Sensor Offset Learning)' '#SF051A_243' 'true' 'REQ:SF051A_243' '' } %GIDa_95506176_73f4_4ba9_b5c7_f4ff23f708dc  Operator=>  OutDataTypeStr=boolean
  ResetHwTqLrng : Subsystem  RequirementInfo={'linktype_rmi_doors' '0000babd (/E-STEER Core/SubSystem Specifications/Application Functions/SF051A Sensor Offset Learning)' '#SF051A_243' 'true' 'REQ:SF051A_243' '' } %GIDa_ec203b45_d0a1_4c9b_964d_3dc0fb0c2020  TreatAsAtomicUnit=on
  Subsystem5 : Subsystem  Description=|  mask(Copyright Information){none=on}
      | Copyright info block.                                               
      |                                                                     
      | Place copyright information at the top of every subsystem in design.
      mask prompts: none "No parameters"
      mask help: Place copyright information at the top of every subsystem in design.
      mask Display:
      | NxtrConf = 'Nexteer Confidential';
      | 
      | sys = bdroot; %handle for the current model ("system")
      | first = get_param(sys,'Created');
      | first = first(end-3:end);  %year is last four digits
      | 
      | last = get_param(sys,'LastModifiedDate');
      | if isempty(last)
      |     last = datestr(now,'yyyy');
      | else
      |     last = last(end-3:end);
      | end
      | 
      | if strcmp(first,last)
      |     fprintf('%s -- Copyright %s Nexteer',NxtrConf,first)
      | else
      |     fprintf('%s -- %s%s- %s Nexteer',NxtrConf,char(169),first,last)
      | end
  wires:
  Constant1/1 -> Relational Operator1/2
  Relational Operator1/1 -> If/1
  SampleCntTot/1 -> Data Type Conversion/1
  If/1 -> ResetHwTqLrng/Action
  Data Type Conversion/1 -> Relational Operator1/1

== system SF051A_SnsrOffsLrng/SnsrOffsLrng/SnsrOffsLrngPer1/Learning/HwPos vs HwTrq Model ==
  note: X2
  note: X1
  note: This block prepares the independent variable for the linear regression --> Y = A1*X1 + A2*X2+ B
      | Where: X1 = sin(HwAg)   nad     X2 = cos(HwAg)
  note: Convert to 3-element array.
  note: The considered mathematical model HwTq vs HwAg follows:
      |                    Y = A*sin(X + Phi) + B
      | Where:
      | -. X = HwAg
      | -. Y = HwTq
      | -. A is the HwTq reading when Tq_Off=0Nm, Phi=0Deg and HwAg=90°
      | -. Phi = HwAg_Offset
      | -. B = HwTq_Offset
      |
      | That model can also be written as:
      |                Y = A1*sin(X) + A2*cos(X) + B
      | Where: A = sqrt(A1^2+A2^2)   and   sin(Phi) = A2/A
      |
      | The RLSE estimates the parameters A1, A2 and B.
  HwAgMeasd : Inport  OutDataTypeStr=single
  Cos_f32 : NxtrMath/Cos_f32  SFunctionSpec=single y1 = Cos_f32(single u1)
      settings: AttributesFormatString=%<MaskType>
  Mux : Mux  Inputs=3
  Row vector : Reshape  OutputDimensionality=Row vector (2-D)  OutputDimensions=[1,3]
  Sin_f32 : NxtrMath/Sin_f32  SFunctionSpec=single y1 = Sin_f32(single u1)
      settings: AttributesFormatString=%<MaskType>
  Subsystem5 : Subsystem  Description=|  mask(Copyright Information){none=on}
      | Copyright info block.                                               
      |                                                                     
      | Place copyright information at the top of every subsystem in design.
      mask prompts: none "No parameters"
      mask help: Place copyright information at the top of every subsystem in design.
      mask Display:
      | NxtrConf = 'Nexteer Confidential';
      | 
      | sys = bdroot; %handle for the current model ("system")
      | first = get_param(sys,'Created');
      | first = first(end-3:end);  %year is last four digits
      | 
      | last = get_param(sys,'LastModifiedDate');
      | if isempty(last)
      |     last = datestr(now,'yyyy');
      | else
      |     last = last(end-3:end);
      | end
      | 
      | if strcmp(first,last)
      |     fprintf('%s -- Copyright %s Nexteer',NxtrConf,first)
      | else
      |     fprintf('%s -- %s%s- %s Nexteer',NxtrConf,char(169),first,last)
      | end
  X0 : Constant  Value=ONE_ULS_F32  OutDataTypeStr=single
      settings: AttributesFormatString=%<OutDataTypeStr>
  constant : Constant  Value=ARCHGLBPRM_PIOVER180_ULS_F32  OutDataTypeStr=single
  deg2rad : Product  Inputs=**  OutDataTypeStr=single
  XAry : Outport
  wires:
  deg2rad/1 -> Sin_f32/1, Cos_f32/1
  constant/1 -> deg2rad/2
  HwAgMeasd/1 -> deg2rad/1
  Row vector/1 -> XAry/1  "TqMdlXAry"
  Mux/1 -> Row vector/1
  X0/1 -> Mux/1
  Cos_f32/1 -> Mux/3  "CosHwAg_HwRadpS_T_f32"
  Sin_f32/1 -> Mux/2  "SinHwAg_HwRadpS_T_f32"

== system SF051A_SnsrOffsLrng/SnsrOffsLrng/SnsrOffsLrngPer1/Learning/Recursive Least Square Regression ==
  note: Note for Coder:
      | In Matlab, a mattrix [3x2] has 3 rows and 2 columns.
      | This notation will be followed inside these blocks  -->
  XAry : Inport
  HwTqMeasd : Inport  Port=2
  Calculate Covariance Matrix : Subsystem
  Calculate K Vector : Subsystem
  Subsystem5 : Subsystem  Description=|  mask(Copyright Information){none=on}
      | Copyright info block.                                               
      |                                                                     
      | Place copyright information at the top of every subsystem in design.
      mask prompts: none "No parameters"
      mask help: Place copyright information at the top of every subsystem in design.
      mask Display:
      | NxtrConf = 'Nexteer Confidential';
      | 
      | sys = bdroot; %handle for the current model ("system")
      | first = get_param(sys,'Created');
      | first = first(end-3:end);  %year is last four digits
      | 
      | last = get_param(sys,'LastModifiedDate');
      | if isempty(last)
      |     last = datestr(now,'yyyy');
      | else
      |     last = last(end-3:end);
      | end
      | 
      | if strcmp(first,last)
      |     fprintf('%s -- Copyright %s Nexteer',NxtrConf,first)
      | else
      |     fprintf('%s -- %s%s- %s Nexteer',NxtrConf,char(169),first,last)
      | end
  Update beta_k : Subsystem
  HwTqOffsEstimd : Outport
  A2 : Outport  Port=2
  wires:
  [X_k] -> Update beta_k/1(XAry)
  XAry/1 -> Calculate K Vector/1(XAry), [X_k]
  Update beta_k/1(HwTqOffsEstimd) -> HwTqOffsEstimd/1
  [X_k] -> Calculate Covariance Matrix/1(XAry)
  HwTqMeasd/1 -> Update beta_k/3(HwTqMeasd)
  Update beta_k/2(A2) -> A2/1
  Calculate K Vector/1(KVect) -> Update beta_k/2(KVect), Calculate Covariance Matrix/2(KVect)

== system SF051A_SnsrOffsLrng/SnsrOffsLrng/SnsrOffsLrngPer1/Learning/Subsystem5 ==

== system SF051A_SnsrOffsLrng/SnsrOffsLrng/SnsrOffsLrngPer1/Learning/Update_NvmRam ==
  HwTqDriftEstimnOnCentr : Inport
  Action Port : ActionPort  ActionType=then
  Constant3 : Constant  RequirementInfo={'linktype_rmi_doors' '0000babd (/E-STEER Core/SubSystem Specifications/Application Functions/SF051A Sensor Offset Learning)' '#SF051A_190' 'true' 'REQ:SF051A_190' '' } %GIDa_6dc44b8d_9f3d_43c8_80fa_fbe50c8cea83  Value=SnsrOffsLrngHwTqOffsLim  OutDataTypeStr=single
  FloatToFixd_s16_f32 : FloatToFixd/FloatToFixd_s16_f32  Param1=12
  LimDyn_f32 : NxtrLim/LimDyn_f32  RequirementInfo={'linktype_rmi_doors' '0000babd (/E-STEER Core/SubSystem Specifications/Application Functions/SF051A Sensor Offset Learning)' '#SF051A_190' 'true' 'REQ:SF051A_190' '' } %GIDa_a95859b7_a762_4c8d_bd03_84d163434d71
  NvmRam : DataStoreWrite  DataStoreName=SnsrOffsLrnd  DataStoreElements=SnsrOffsLrnd.HwTqOffs
  Subsystem5 : Subsystem  Description=|  mask(Copyright Information){none=on}
      | Copyright info block.                                               
      |                                                                     
      | Place copyright information at the top of every subsystem in design.
      mask prompts: none "No parameters"
      mask help: Place copyright information at the top of every subsystem in design.
      mask Display:
      | NxtrConf = 'Nexteer Confidential';
      | 
      | sys = bdroot; %handle for the current model ("system")
      | first = get_param(sys,'Created');
      | first = first(end-3:end);  %year is last four digits
      | 
      | last = get_param(sys,'LastModifiedDate');
      | if isempty(last)
      |     last = datestr(now,'yyyy');
      | else
      |     last = last(end-3:end);
      | end
      | 
      | if strcmp(first,last)
      |     fprintf('%s -- Copyright %s Nexteer',NxtrConf,first)
      | else
      |     fprintf('%s -- %s%s- %s Nexteer',NxtrConf,char(169),first,last)
      | end
  Unary Minus : UnaryMinus  RequirementInfo={'linktype_rmi_doors' '0000babd (/E-STEER Core/SubSystem Specifications/Application Functions/SF051A Sensor Offset Learning)' '#SF051A_190' 'true' 'REQ:SF051A_190' '' } %GIDa_a7123fff_4a4e_4e7a_bbb1_3e64357493ac
  wires:
  HwTqDriftEstimnOnCentr/1 -> LimDyn_f32/1
  LimDyn_f32/1 -> FloatToFixd_s16_f32/1
  FloatToFixd_s16_f32/1 -> NvmRam/1
  Unary Minus/1 -> LimDyn_f32/2
  Constant3/1 -> LimDyn_f32/3, Unary Minus/1

== system SF051A_SnsrOffsLrng/SnsrOffsLrng/SnsrOffsLrngPer1/Learning/ValidityCheck ==
  note: The logic for CntTot>0 has been removed to avoid coverage issues.
      | The Signal CntTot is the addition of CntPos + CntNeg.
      | The block "Decide Outputs" contains a calculation were
      | CntTot is dividing.
      | This block will only be executed when CntPos AND CntNeg are
      | bigger than zero, which means that CntTot is also bigger than zero.
  note: EstimationValid
      | 0 = HwTrq NotLearned
      | 1 = HwTrq Offset Learned
  note: TOCStatus
      | 0 = HwTrq NotLearned
      | 1 = Positive HwTrq Offset
      | 2 = Negative HwTrqOffset
      | 3 = Zero HwTrq Offset
      | 4 = HwTrq Offset Learned
  SampleCntTot : Inport
  SampleCntPos : Inport  Port=2
  SampleCntNeg : Inport  Port=3
  HwTqDriftEstimnOnCentr : Inport  Port=4
  Constant1 : Constant  Value=0  OutDataTypeStr=uint16
      settings: AttributesFormatString=%<OutDataTypeStr>
  Constant2 : Constant  Value=0  OutDataTypeStr=uint16
      settings: AttributesFormatString=%<OutDataTypeStr>
  DecideOutputs : Subsystem
  Display : DataStoreWrite  DataStoreName=dSnsrOffsLrngHwTqLrngEstimnVldt
  HwTrqNotLearnt : Subsystem  TreatAsAtomicUnit=on
  If : If  NumInputs=2  IfExpression=u1&u2
  Merge : Merge
  Merge1 : Merge
  NvmRam : DataStoreWrite  DataStoreName=SnsrOffsLrnd  DataStoreElements=SnsrOffsLrnd.HwTqLrngSts
  Relational Operator1 : RelationalOperator  Operator=>  OutDataTypeStr=boolean
  Relational Operator6 : RelationalOperator  Operator=>  OutDataTypeStr=boolean
  Subsystem5 : Subsystem  Description=|  mask(Copyright Information){none=on}
      | Copyright info block.                                               
      |                                                                     
      | Place copyright information at the top of every subsystem in design.
      mask prompts: none "No parameters"
      mask help: Place copyright information at the top of every subsystem in design.
      mask Display:
      | NxtrConf = 'Nexteer Confidential';
      | 
      | sys = bdroot; %handle for the current model ("system")
      | first = get_param(sys,'Created');
      | first = first(end-3:end);  %year is last four digits
      | 
      | last = get_param(sys,'LastModifiedDate');
      | if isempty(last)
      |     last = datestr(now,'yyyy');
      | else
      |     last = last(end-3:end);
      | end
      | 
      | if strcmp(first,last)
      |     fprintf('%s -- Copyright %s Nexteer',NxtrConf,first)
      | else
      |     fprintf('%s -- %s%s- %s Nexteer',NxtrConf,char(169),first,last)
      | end
  LrngSts : Outport
  EstimnVld : Outport  Port=2
  wires:
  SampleCntNeg/1 -> [SampleCntNeg], Relational Operator6/1
  Constant2/1 -> Relational Operator6/2
  SampleCntPos/1 -> [SampleCntPos], Relational Operator1/1
  Relational Operator1/1 -> If/1
  Relational Operator6/1 -> If/2
  Constant1/1 -> Relational Operator1/2
  [SampleCntPos] -> DecideOutputs/1(CntPos)
  [SampleCntNeg] -> DecideOutputs/2(CntNeg)
  SampleCntTot/1 -> DecideOutputs/3(CntTot)
  HwTqDriftEstimnOnCentr/1 -> DecideOutputs/4(DriftEstimnOnCentr)
  DecideOutputs/1(LrngSts) -> Merge/1
  DecideOutputs/2(EstimnVld) -> Merge1/1
  If/1 -> DecideOutputs/Action
  Merge/1 -> LrngSts/1, NvmRam/1
  Merge1/1 -> Display/1, EstimnVld/1
  If/2 -> HwTrqNotLearnt/Action
  HwTrqNotLearnt/1(LrngSts) -> Merge/2
  HwTrqNotLearnt/2(EstimnVld) -> Merge1/2
